simulink library "PC_Simulator_Lib"  (Simulink 8.2)
settings: Solver=ode45  StartTime=0.0  StopTime=10.0  RelTol=1e-3
values from neighbouring files (symbols this model uses):
  data = [r1 r2 r3 r4 L1 L2 L3 L4]    [strasse_Bedatung_HNI_ITI.m]
  distSameLane = 60    [InitialisationsEnv.m]
  eng_speed = [0 60 120 180 240 300 360 420 480 540 600 660 ... (101 elements, 1x101)]    [engine_table.mat]    (also in motor_parameter_calc.m = omega)
  Heading_init = 0    [Start.m]
  inertiaLateral = 25*(radiusWheel)^2    (= 4.129024)    [Start.m]
  laneWidth = 3.6    [InitialisationsEnv.m]    (also in strasse_Bedatung_HNI_ITI.m)
  omega_engine = [0.000000 150.000000 500.000000 1000.000000 1500.000000 2000.000000 2500.000000 3000.000000 3500.000000 4000.000000 4500.000000 5000.000000 5500.000000 6000.000000]    [friction_tables.m]
  omega_max = 6000    [engine_table.mat]    (also in motor_parameter_calc.m)
  omega_wheel = [0 20 40 60 80 100 122 143.7 164]    [friction_tables.m]
  para_Fellow_8_Points = ADAS.Fellow_8_Points    [ADAS_parameters.m]
  position_start_x = [x1 x2 x3 x4 x5 x6 x7]    [strasse_Bedatung_HNI_ITI.m]
  position_start_y = [y1 y2 y3 y4 y5 y6 y7]    [strasse_Bedatung_HNI_ITI.m]
  rad3rdLine = 57.2    [InitialisationsEnv.m]    (also in strasse_Bedatung_HNI_ITI.m)
  radiusWheel = 16*2.54/100    (= 0.4064)    [Start.m]
  s_values = [S1 S2 S3 S4 S5 S6 S7]    [strasse_Bedatung_HNI_ITI.m]
  segmentLimits = [segment1EndThirdLine                   segment2EndThirdLine                   segment3EndThirdLine                   segment4EndThirdLine                   segment5EndThirdLine                   segment6EndThirdLine                   segment7EndThirdLine                   segment8EndThirdLine                   ]    [InitialisationsEnv.m]    (also in strasse_Bedatung_HNI_ITI.m)
  setPosT = [-1.8 -5.4 -1.8 -5.4 -1.8 -5.4 -1.8 -5.4 -1.8 -5.4]    [InitialisationsEnv.m]
  torque = [297.089227105 300.997600937 304.800343044 308.497453426 312.088932082 315.574779014 318.95499422 322.229577701 325.398529457 328.461849487 331.419537793 334.271594373 ... (101 elements, 1x101)]    [engine_table.mat]    (also in motor_parameter_calc.m = g)
  Torque_lost = [0.000000 -8.777780 -15.000000 -26.800000 -29.600000 -32.700000 -35.900000 -39.300000 -42.800000 -46.500000 -50.300000 -54.300000 -58.500000 -62.800000 ]*0.6    [friction_tables.m]
  Torque_lost_wheel = [0.8 0.8 0.75 0.7 0.4 0.3 0.2 0.07 0.07]*0.2    [friction_tables.m]
  X_init = 0    [Start.m]
  Y_init = 1.8    [Start.m]
  Z_init = 0    [Start.m]
undefined symbols (not defined in the file or in its folder): Acc_Pedal, ADAS, Brake_Pedal, Joystick, Newton, Para, Raphson, Standard_Devices, Steering_Wheel_Angle, UDP_Protocol
libraries: simulink x43, rtwinlib x7, dspnetwork x2, simulink_extras x1, vrlib x1
(part 8 of 13)

== system PC_Simulator_Lib/Vehicle dynamics/velocity/to_tire ==
  angel_of_rotation_of_front_left_wheel : Inport
  angel_of_rotation_of_front_Right_wheel : Inport  Port=2
  velocity_at_wheels_in_X_mux(4) : Inport  Port=3
  velocity_at_wheels_in_Y_mux(4) : Inport  Port=4
  Demux : Demux
  Demux1 : Demux
  La{,1..7} (8 alike) : Product  RndMeth=Zero
  Mux1 : Mux
  Mux6 : Mux
  Sum1 : Sum  Inputs=+-
  Sum2 : Sum
  Sum3 : Sum  Inputs=+-
  Sum4 : Sum
  T1 : Trigonometry
  T2 : Trigonometry  Operator=cos
  T3 : Trigonometry  Operator=cos
  T4 : Trigonometry
  velocity_at_wheels_in_X_mux(4)final : Outport
  velocity_at_wheels_in_Y_mux(4)final : Outport  Port=2
  wires:
  velocity_at_wheels_in_X_mux(4)/1 -> Demux/1
  velocity_at_wheels_in_Y_mux(4)/1 -> Demux1/1
  Demux/3 -> Mux6/3
  Demux/4 -> Mux6/4
  Demux1/3 -> Mux1/3
  Demux1/4 -> Mux1/4
  Mux6/1 -> velocity_at_wheels_in_X_mux(4)final/1
  Mux1/1 -> velocity_at_wheels_in_Y_mux(4)final/1
  angel_of_rotation_of_front_left_wheel/1 -> T2/1, T4/1
  angel_of_rotation_of_front_Right_wheel/1 -> T3/1, T1/1
  Demux/1 -> La/1, La3/1, La4/1
  T2/1 -> La2/2, La/2
  La/1 -> Sum4/1
  Demux1/1 -> La2/1, La1/1
  T4/1 -> La3/2, La1/2
  La1/1 -> Sum4/2
  Sum4/1 -> Mux6/1
  La4/1 -> Sum2/1
  La7/1 -> Sum2/2
  Sum2/1 -> Mux6/2
  Demux1/2 -> La5/1, La7/1
  La2/1 -> Sum3/1
  La3/1 -> Sum3/2
  Sum3/1 -> Mux1/1
  La5/1 -> Sum1/1
  La6/1 -> Sum1/2
  Sum1/1 -> Mux1/2
  T3/1 -> La5/2, La4/2
  Demux/2 -> La6/1
  T1/1 -> La6/2, La7/2

== system PC_Simulator_Lib/Vehicle dynamics/velocity/velocity_at_Front_Left ==
  rate_of_change_Yaw_Angle : Inport
  longitudenal_velocity_Vx : Inport  Port=2
  Lateral_velocity_Vy : Inport  Port=3
  Divide : Product  Inputs=*/
  Length_CG_Front_Wheels : Constant  Value=Para.VD.Length_Front.v
  Product : Product  RndMeth=Zero
  Product1 : Product  RndMeth=Zero
  Rfl : Math  Operator=sqrt  SaturateOnIntegerOverflow=on
  Sum : Sum  Inputs=|++
  Sum1 : Sum  Inputs=|++
  Sum2 : Sum  Inputs=|++
  Sum3 : Sum  Inputs=|-+
  T1 : Trigonometry  Operator=cos
  T2 : Trigonometry
  ThetaFl : Trigonometry  Operator=atan
  Vfl/CG : Product  RndMeth=Zero
  Vfr/CGx : Product  RndMeth=Zero
  Vfr/CGy : Product  RndMeth=Zero
  Width_of_Car/2 : Constant  Value=Para.VD.Wheel_Base_Width.v/2
  pi : Constant  Value=pi
  velocity_at_Front_left_in_X : Outport
  velocity_at_Front_left_in_Y : Outport  Port=2
  wires:
  Lateral_velocity_Vy/1 -> Sum2/2
  Sum2/1 -> velocity_at_Front_left_in_Y/1
  longitudenal_velocity_Vx/1 -> Sum1/2
  Sum1/1 -> velocity_at_Front_left_in_X/1
  rate_of_change_Yaw_Angle/1 -> Vfl/CG/2
  Sum/1 -> Rfl/1
  Product/1 -> Sum/1
  Length_CG_Front_Wheels/1 -> Divide/1, Product/2, Product/1
  Width_of_Car/2/1 -> Divide/2, Product1/2, Product1/1
  Product1/1 -> Sum/2
  Rfl/1 -> Vfl/CG/1
  Divide/1 -> ThetaFl/1
  ThetaFl/1 -> Sum3/1
  Vfl/CG/1 -> Vfr/CGy/1, Vfr/CGx/1
  T2/1 -> Vfr/CGy/2
  T1/1 -> Vfr/CGx/2
  Sum3/1 -> T2/1, T1/1
  Vfr/CGx/1 -> Sum1/1
  Vfr/CGy/1 -> Sum2/1
  pi/1 -> Sum3/2

== system PC_Simulator_Lib/Vehicle dynamics/velocity/velocity_at_Front_Right ==
  rate_of_change_Yaw_Angle : Inport
  longitudenal_velocity_Vx : Inport  Port=2
  Lateral_velocity_Vy : Inport  Port=3
  Divide : Product  Inputs=*/
  Length_CG_Front_Wheels : Constant  Value=Para.VD.Length_Front.v
  Product : Product  RndMeth=Zero
  Product1 : Product  RndMeth=Zero
  Rfr : Math  Operator=sqrt  SaturateOnIntegerOverflow=on
  Sum : Sum  Inputs=|++
  Sum1 : Sum  Inputs=|++
  Sum2 : Sum  Inputs=|++
  ThetaFr : Trigonometry  Operator=atan
  ThetaFr1 : Trigonometry  Operator=cos
  ThetaFr2 : Trigonometry
  Vfr/CG : Product  RndMeth=Zero
  Vfr/CG1 : Product  RndMeth=Zero
  Vfr/CG2 : Product  RndMeth=Zero
  Width_of_Car/2 : Constant  Value=Para.VD.Wheel_Base_Width.v/2
  sign : Gain
  velocity_at_Front_Right_in_X : Outport
  velocity_at_Front_Right_in_Y : Outport  Port=2
  wires:
  Vfr/CG2/1 -> Sum2/1
  Vfr/CG1/1 -> Sum1/1
  sign/1 -> ThetaFr1/1, ThetaFr2/1
  ThetaFr1/1 -> Vfr/CG1/2
  ThetaFr2/1 -> Vfr/CG2/2
  Vfr/CG/1 -> Vfr/CG1/1, Vfr/CG2/1
  ThetaFr/1 -> sign/1
  Divide/1 -> ThetaFr/1
  Rfr/1 -> Vfr/CG/1
  Product1/1 -> Sum/2
  Width_of_Car/2/1 -> Product1/1, Product1/2, Divide/2
  Length_CG_Front_Wheels/1 -> Product/1, Product/2, Divide/1
  Product/1 -> Sum/1
  Sum/1 -> Rfr/1
  rate_of_change_Yaw_Angle/1 -> Vfr/CG/2
  Sum1/1 -> velocity_at_Front_Right_in_X/1
  longitudenal_velocity_Vx/1 -> Sum1/2
  Sum2/1 -> velocity_at_Front_Right_in_Y/1
  Lateral_velocity_Vy/1 -> Sum2/2

== system PC_Simulator_Lib/Vehicle dynamics/velocity/velocity_at_Rear_Left ==
  rate_of_change_Yaw_Angle : Inport
  longitudenal_velocity_Vx : Inport  Port=2
  Lateral_velocity_Vy : Inport  Port=3
  Divide : Product  Inputs=*/
  Divide1 : Product  Inputs=*/
  Length_CG_Rear_Wheels : Constant  Value=Para.VD.Length_Rear.v
  Product : Product  RndMeth=Zero
  Product1 : Product  RndMeth=Zero
  Rrl : Math  Operator=sqrt  SaturateOnIntegerOverflow=on
  Sum{,1..3} (4 alike) : Sum  Inputs=|++
  T1 : Trigonometry  Operator=cos
  T2 : Trigonometry
  Thetarl : Trigonometry  Operator=atan
  Vrl/CG : Product  RndMeth=Zero
  Vrl/CGx : Product  RndMeth=Zero
  Vrl/CGy : Product  RndMeth=Zero
  Width_of_Car/2 : Constant  Value=Para.VD.Wheel_Base_Width.v/2
  pi : Constant  Value=pi
  s : Trigonometry  Operator=atan
  velocity_at_Rear_left_in_X : Outport
  velocity_at_Rear_left_in_Y : Outport  Port=2
  slip_angel_at_Rear_left : Outport  Port=3
  wires:
  Vrl/CGy/1 -> Sum2/1
  Vrl/CGx/1 -> Sum1/1
  Sum3/1 -> T1/1, T2/1
  T1/1 -> Vrl/CGx/2
  T2/1 -> Vrl/CGy/2
  Vrl/CG/1 -> Vrl/CGx/1, Vrl/CGy/1
  Thetarl/1 -> Sum3/1
  Divide/1 -> Thetarl/1
  Rrl/1 -> Vrl/CG/1
  Product1/1 -> Sum/2
  Width_of_Car/2/1 -> Product1/1, Product1/2, Divide/2
  Length_CG_Rear_Wheels/1 -> Product/1, Product/2, Divide/1
  Product/1 -> Sum/1
  Sum/1 -> Rrl/1
  rate_of_change_Yaw_Angle/1 -> Vrl/CG/2
  Sum1/1 -> Divide1/2, velocity_at_Rear_left_in_X/1
  longitudenal_velocity_Vx/1 -> Sum1/2
  Sum2/1 -> Divide1/1, velocity_at_Rear_left_in_Y/1
  Lateral_velocity_Vy/1 -> Sum2/2
  pi/1 -> Sum3/2
  Divide1/1 -> s/1
  s/1 -> slip_angel_at_Rear_left/1

== system PC_Simulator_Lib/Vehicle dynamics/velocity/velocity_at_Rear_Right ==
  rate_of_change_Yaw_Angle : Inport
  longitudenal_velocity_Vx : Inport  Port=2
  Lateral_velocity_Vy : Inport  Port=3
  Divide : Product  Inputs=*/
  Length_CG_Rear_Wheels : Constant  Value=Para.VD.Length_Rear.v
  Product : Product  RndMeth=Zero
  Product1 : Product  RndMeth=Zero
  Rrr : Math  Operator=sqrt  SaturateOnIntegerOverflow=on
  Sum : Sum  Inputs=|++
  Sum1 : Sum  Inputs=|++
  Sum2 : Sum  Inputs=|++
  T1 : Trigonometry  Operator=cos
  T2 : Trigonometry
  Thetarr : Trigonometry  Operator=atan
  Vrr/CG : Product  RndMeth=Zero
  Vrr/CGx : Product  RndMeth=Zero
  Vrr/CGy : Product  RndMeth=Zero
  Width_of_Car/2 : Constant  Value=Para.VD.Wheel_Base_Width.v/2
  sign : Gain  Gain=-1
  velocity_at_Rear_Right_in_X : Outport
  velocity_at_Rear_Right_in_Y : Outport  Port=2
  wires:
  Lateral_velocity_Vy/1 -> Sum2/2
  Sum2/1 -> velocity_at_Rear_Right_in_Y/1
  longitudenal_velocity_Vx/1 -> Sum1/2
  Sum1/1 -> velocity_at_Rear_Right_in_X/1
  rate_of_change_Yaw_Angle/1 -> Vrr/CG/2
  Sum/1 -> Rrr/1
  Product/1 -> Sum/1
  Length_CG_Rear_Wheels/1 -> Divide/1, Product/2, Product/1
  Width_of_Car/2/1 -> Divide/2, Product1/2, Product1/1
  Product1/1 -> Sum/2
  Rrr/1 -> Vrr/CG/1
  Divide/1 -> Thetarr/1
  Thetarr/1 -> sign/1
  Vrr/CG/1 -> Vrr/CGy/1, Vrr/CGx/1
  T2/1 -> Vrr/CGy/2
  T1/1 -> Vrr/CGx/2
  sign/1 -> T2/1, T1/1
  Vrr/CGx/1 -> Sum1/1
  Vrr/CGy/1 -> Sum2/1

== system PC_Simulator_Lib/Vehicle dynamics/velocity/velocity_conditioning ==
  velocity_at_wheels_in_X_mux(4)in : Inport
  velocity_at_wheels_in_Y_mux(4)in : Inport  Port=2
  R_CGin : Inport  Port=3
  VxCG : Inport  Port=4
  VyCG : Inport  Port=5
  Constant1 : Constant  Value=eps
  Constant3 : Constant  Value=0
  Constant4 : Constant  Value=0
  Constant5 : Constant  Value=inf
  Demux : Demux
  Demux1 : Demux
  Logical Operator : Logic  Operator=NOT  AllPortsSameDT=off  OutDataTypeStr=boolean
  Logical Operator1 : Logic  Operator=OR  AllPortsSameDT=off  OutDataTypeStr=boolean
  Mux{1,4..6} (4 alike) : Mux
  Relational Operator1 : RelationalOperator  Operator===  OutDataTypeStr=boolean
  Relational Operator2 : RelationalOperator  Operator===  OutDataTypeStr=boolean
  Sum2 : Sum  Inputs=|++
  Switch1 : Switch
  Switch2 : Switch
  Switch3 : Switch
  Velocitytrim : Subsystem
  Velocitytrim1 : Subsystem
  Velocitytrim2 : Subsystem
  Velocitytrim3 : Subsystem
  Velocitytrim4 : Subsystem
  Velocitytrim5 : Subsystem
  Velocitytrim6 : Subsystem
  Velocitytrim7 : Subsystem
  velocity_at_wheels_in_X_mux(4)out : Outport
  velocity_at_wheels_in_Y_mux(4)out : Outport  Port=2
  R_CGout : Outport  Port=3
  wires:
  Constant3/1 -> Relational Operator1/2
  Constant4/1 -> Relational Operator2/2
  Relational Operator1/1 -> Logical Operator1/1
  Relational Operator2/1 -> Logical Operator1/2
  Mux5/1 -> Switch1/3
  Mux4/1 -> Switch2/3
  Constant5/1 -> Switch3/3
  Logical Operator/1 -> Switch1/2, Switch2/2, Switch3/2
  Logical Operator1/1 -> Logical Operator/1
  Switch3/1 -> Sum2/1
  Constant1/1 -> Sum2/2
  VxCG/1 -> Mux5/1, Mux5/2, Mux5/3, Mux5/4, Relational Operator1/1
  VyCG/1 -> Relational Operator2/1, Mux4/1, Mux4/2, Mux4/3, Mux4/4
  velocity_at_wheels_in_X_mux(4)in/1 -> Switch1/1
  velocity_at_wheels_in_Y_mux(4)in/1 -> Switch2/1
  R_CGin/1 -> Switch3/1
  Sum2/1 -> R_CGout/1
  Demux/1 -> Velocitytrim/1(vin)
  Demux/2 -> Velocitytrim1/1(vin)
  Demux/3 -> Velocitytrim2/1(vin)
  Demux/4 -> Velocitytrim3/1(vin)
  Velocitytrim/1(vout) -> Mux6/1
  Velocitytrim1/1(vout) -> Mux6/2
  Velocitytrim2/1(vout) -> Mux6/3
  Velocitytrim3/1(vout) -> Mux6/4
  Switch1/1 -> Demux/1
  Mux6/1 -> velocity_at_wheels_in_X_mux(4)out/1
  Demux1/1 -> Velocitytrim4/1(vin)
  Demux1/2 -> Velocitytrim5/1(vin)
  Demux1/3 -> Velocitytrim6/1(vin)
  Demux1/4 -> Velocitytrim7/1(vin)
  Velocitytrim4/1(vout) -> Mux1/1
  Velocitytrim5/1(vout) -> Mux1/2
  Velocitytrim6/1(vout) -> Mux1/3
  Velocitytrim7/1(vout) -> Mux1/4
  Mux1/1 -> velocity_at_wheels_in_Y_mux(4)out/1
  Switch2/1 -> Demux1/1

== system PC_Simulator_Lib/ADAS/Decision_Making_ADAS/Decision_Unit/critical_Braking_distance_determination ==
  v_relative_Sensor[m|s] : Inport
  1-D Lookup Table1 : Lookup_n-D  NumberOfTableDimensions=1  BreakpointsForDimension1=ADAS.EBA.Braking_Distance_LookUpTable.velocity  BeginIndexSearchUsingPreviousIndexResult=on  Table=ADAS.EBA.Braking_Distance_LookUpTable.Distance  InternalRulePriority=Speed  RndMeth=Simplest  InputSameDT=on
  Abs : Abs
  Divide : Product  Inputs=/**
  Gain : Gain  Gain=3.6
  Math Function : Math  Operator=square  SaturateOnIntegerOverflow=on
  Sign : Signum
  Unary Minus : UnaryMinus
  Braking_Distance[m] : Outport
  wires:
  v_relative_Sensor[m|s]/1 -> Abs/1, Sign/1, Math Function/1
  Math Function/1 -> Divide/2
  Divide/1 -> Braking_Distance[m]/1
  Gain/1 -> 1-D Lookup Table1/1
  1-D Lookup Table1/1 -> Divide/1
  Abs/1 -> Gain/1
  Sign/1 -> Unary Minus/1
  Unary Minus/1 -> Divide/3

== system PC_Simulator_Lib/ADAS/Decision_Making_ADAS/Maping_Input/signals_manipulation ==
  ACC_State : Inport
  Pilotiertes_Fahren_State : Inport  Port=2
  Emergency_Brkae_State : Inport  Port=3
  Emergency_Steering_State : Inport  Port=4
  Add : Sum  Inputs=++++
  Gain : Gain
  Gain1 : Gain  Gain=2
  Gain2 : Gain  Gain=3
  Gain3 : Gain  Gain=4
  Memory{1..4} (4 alike) : Memory
  Active_System : Outport
  wires:
  ACC_State/1 -> Memory1/1
  Pilotiertes_Fahren_State/1 -> Memory2/1
  Memory1/1 -> Gain/1
  Memory2/1 -> Gain1/1
  Add/1 -> Active_System/1
  Gain/1 -> Add/1
  Gain1/1 -> Add/2
  Emergency_Brkae_State/1 -> Memory3/1
  Memory3/1 -> Gain2/1
  Gain2/1 -> Add/3
  Gain3/1 -> Add/4
  Memory4/1 -> Gain3/1
  Emergency_Steering_State/1 -> Memory4/1

== system PC_Simulator_Lib/ADAS/Decision_Making_ADAS/Trajectory_calculatin_and_distance_control_and output_maping/Calculate_Desired_Trajectory ==
  Enable_Lateral_Controller : Inport
  T_Desired_initial[m] : Inport  Port=2
  Delta_T_Rate_limitl[m|s] : Inport  Port=3
  x[m] : Inport  Port=4
  y[m] : Inport  Port=5
  Yaw_Angle[rad] : Inport  Port=6
  Vx_CoG[m|s] : Inport  Port=7
  Velocity_Desired[m|s] : Inport  Port=8
  Bus Creator1 : BusCreator  Inputs=6
  Curvature_Calculation : Subsystem
  Gain{,1..5} (6 alike) : Gain
  Gain6 : Gain  Gain=pi/180
  Ground : Ground
  Road model ST_XY : Subsystem  Description=Simple road model to transform the (s,t) point of the local coordinate system to (x,y) point of the global coordinate system
  Scope1 : Scope
      settings: SaveName=ScopeData18
  Scope2 : Scope
  Scope3 : Scope  NumInputPorts=3
      settings: YMin=-5~-5~-5  YMax=5~5~5
  Strasse_xy : Subsystem
  Terminator : Terminator
  adding_Delta_s_and_road_restart : Subsystem
  applying_Desired_T_Gradually : Subsystem
  x_y_Virtual_Point_Calculation : Subsystem
  Desired_Track : Outport
  tag scope: T_VP=global
  wires:
  Bus Creator1/1 -> Desired_Track/1
  Gain3/1 -> Bus Creator1/4  "acceleration_Desired[m|s2]"
  Gain1/1 -> Bus Creator1/2  "y_Desired[m]"
  Gain4/1 -> Bus Creator1/5  "Heading_angle_Desired[rad]"
  Gain/1 -> Bus Creator1/1  "x_Desired[m]"
  Gain2/1 -> Bus Creator1/3  "Velocity_Desired[m|s]"
  Gain5/1 -> Bus Creator1/6  "Curvature_Desired_Track[1|m]"
  Gain6/1 -> Gain4/1
  Curvature_Calculation/1(Curvature_Given_Point[1|m]) -> Gain5/1
  x_y_Virtual_Point_Calculation/1(x_Virtual_Point[m]) -> Strasse_xy/1(x[m])
  x_y_Virtual_Point_Calculation/2(y_Virtual_Point[m]) -> Strasse_xy/2(y[m])
  Strasse_xy/1(s[m]) -> adding_Delta_s_and_road_restart/1(S_Virtual_Point_Actual[m])
  applying_Desired_T_Gradually/1(T_Desired_execute[m]) -> Scope1/1, Scope3/3, Road model ST_XY/2(t[m]), Curvature_Calculation/2(t_Value[m])
  adding_Delta_s_and_road_restart/1(S_Virtual_Point_Desired[m]) -> Road model ST_XY/1(s[m])
  Road model ST_XY/1(x[m]) -> Gain/1
  Road model ST_XY/2(y[m]) -> Gain1/1
  Road model ST_XY/3(headingAngle[deg]) -> Gain6/1
  Road model ST_XY/4(curvature[1/m]) -> Curvature_Calculation/1(Curvature_Road_Center[1|m])
  Strasse_xy/3(Heading_angle[rad]) -> Terminator/1
  Ground/1 -> Gain3/1
  Enable_Lateral_Controller/1 -> applying_Desired_T_Gradually/1(Enable_Lateral_Controller)
  T_Desired_initial[m]/1 -> applying_Desired_T_Gradually/3(T_Desired_initial[m]), Scope2/1, Scope3/2
  Delta_T_Rate_limitl[m|s]/1 -> applying_Desired_T_Gradually/4(Delta_T_Rate_limitl[m|s])
  Velocity_Desired[m|s]/1 -> Gain2/1
  Strasse_xy/2(t[m]) -> [T_VP], applying_Desired_T_Gradually/2(T_current[m]), Scope3/1
  Yaw_Angle[rad]/1 -> x_y_Virtual_Point_Calculation/3(Yaw_Angle[rad])
  x[m]/1 -> x_y_Virtual_Point_Calculation/1(x[m])
  y[m]/1 -> x_y_Virtual_Point_Calculation/2(y[m])
  Vx_CoG[m|s]/1 -> applying_Desired_T_Gradually/5(Vx_CoG[m|s]), adding_Delta_s_and_road_restart/2(Vx_CoG[m|s])

== system PC_Simulator_Lib/ADAS/Decision_Making_ADAS/Trajectory_calculatin_and_distance_control_and output_maping/Distance_Control ==
  Parameter_Bus : Inport
  Distance_2_Felow_Vehicle[m] : Inport  Port=2
  V_realtive[m|s] : Inport  Port=3
  V_Vehicle[m|s] : Inport  Port=4
  Time_Gap[s] : Inport  Port=5
  V_User_Set_Speed[m|s] : Inport  Port=6
  Enable : EnablePort
  Bus Selector : BusSelector  OutputSignals=acceleration_min[m|s2]
  Bus Selector1 : BusSelector  OutputSignals=V_Desired_max[m|s],V_Desired_min[m|s]
  Calculate_distances : Subsystem
  Distance controller : Subsystem
  V_Desired_Following[m|s] : Outport
  wires:
  V_Vehicle[m|s]/1 -> Distance controller/5(V_Vehicle[m|s]), Calculate_distances/3(V_Vehicle[m|s])
  Time_Gap[s]/1 -> Calculate_distances/4(Time_Gap_Desired[s])
  V_realtive[m|s]/1 -> Distance controller/4(V_realtive[m|s]), Calculate_distances/2(V_realtive[m|s])
  Distance controller/1(V_Desired_Following[m|s]) -> V_Desired_Following[m|s]/1
  Calculate_distances/1(S_Start_Braking[m]) -> Distance controller/2(S_Start_Braking[m])
  Distance_2_Felow_Vehicle[m]/1 -> Distance controller/1(Distance_2_Felow_Vehicle[m])
  Calculate_distances/2(Distance_Desired[m]) -> Distance controller/3(Distance_desired[m])
  Parameter_Bus/1 -> Bus Selector1/1, Bus Selector/1
  Bus Selector/1 -> Calculate_distances/1(acceleration_min[m|s2])  "<acceleration_min[m|s2]>"
  Bus Selector1/2 -> Distance controller/7(V_Desired_min[m|s])  "<V_Desired_min[m|s]>"
  Bus Selector1/1 -> Distance controller/6(V_Desired_max[m|s])  "<V_Desired_max[m|s]>"
  V_User_Set_Speed[m|s]/1 -> Distance controller/8(V_User_Set_Speed[m|s])

== system PC_Simulator_Lib/ADAS/Decision_Making_ADAS/Trajectory_calculatin_and_distance_control_and output_maping/Parameters ==
  Bus Creator : BusCreator
  Constant1 : Constant  Value=ADAS.Velocity_Control.a_min
  Constant2 : Constant  Value=200/3.6
  Constant3 : Constant  Value=0/3.6
  Constant4 : Constant  Value=ADAS.Velocity_Control.a_max
  Out1 : Outport
  wires:
  Bus Creator/1 -> Out1/1  "ADAS_Parameters"
  Constant4/1 -> Bus Creator/1  "acceleration_max[m|s2]"
  Constant1/1 -> Bus Creator/2  "acceleration_min[m|s2]"
  Constant2/1 -> Bus Creator/3  "V_Desired_max[m|s]"
  Constant3/1 -> Bus Creator/4  "V_Desired_min[m|s]"

== system PC_Simulator_Lib/ADAS/Execution_ADAS/Lateral_Controller_S_Function/Lateral_controller ==
  x_CoG_Global : Inport
  y_CoG_Global : Inport  Port=2
  v_CoG : Inport  Port=3
  Slip_Angle : Inport  Port=4
  Yaw_Angle : Inport  Port=5
  Yaw_Rate : Inport  Port=6
  x_Desire : Inport  Port=7
  y_Desired : Inport  Port=8
  Yaw_Desired : Inport  Port=9
  Yaw_Rate_Desired : Inport  Port=10
  v_Desired : Inport  Port=11
  a_Desired : Inport  Port=12
  Gain18 : Gain  Gain=-1
  Inverse_Steering_system : Subsystem
  control_law : Subsystem
  Steering_Wheel_Angle[norm] : Outport
  wires:
  Gain18/1 -> control_law/4(Slip_Angle)
  x_CoG_Global/1 -> control_law/1(x_CoG_Global)
  y_CoG_Global/1 -> control_law/2(y_CoG_Global)
  a_Desired/1 -> control_law/12(a_Desired)
  v_Desired/1 -> control_law/11(v_Desired)
  v_CoG/1 -> control_law/3(v_CoG)
  Yaw_Rate_Desired/1 -> control_law/10(Yaw_Rate_Desired)
  Slip_Angle/1 -> Gain18/1
  Yaw_Desired/1 -> control_law/9(Yaw_Desired)
  Yaw_Angle/1 -> control_law/5(Yaw_Angle)
  y_Desired/1 -> control_law/8(y_Desired)
  Yaw_Rate/1 -> control_law/6(Yaw_Rate)
  x_Desire/1 -> control_law/7(x_Desire)
  control_law/1(Inner_Wheel_Steeringangle[rad]) -> Inverse_Steering_system/1(Inner_Wheel_Steeringangle[rad])
  Inverse_Steering_system/1(Steering_Wheel_Angle[norm]) -> Steering_Wheel_Angle[norm]/1

== system PC_Simulator_Lib/ADAS/Execution_ADAS/Lateral_Controller_S_Function/calculate_slip_ange_and_absolute_velocity ==
  Vx_CoG[m|s] : Inport
  Vy_CoG[m|s] : Inport  Port=2
  Add : Sum
  Add1 : Sum
  Compare To Constant1 : simulink/Logic and Bit Operations/Compare To Constant  relop=>=  const=1  OutDataTypeStr=boolean
  Constant : Constant  Value=eps
  Data Type Conversion : DataTypeConversion
  Math Function : Math  Operator=square  SaturateOnIntegerOverflow=on
  Math Function1 : Math  Operator=square  SaturateOnIntegerOverflow=on
  Product1 : Product
  Sqrt : Sqrt  AlgorithmType=Newton-Raphson  SaturateOnIntegerOverflow=on
  Trigonometric Function : Trigonometry  Operator=atan2
  v_CoG[m|s] : Outport
  Slip_Angle[rad] : Outport  Port=2
  wires:
  Constant/1 -> Add1/2
  Sqrt/1 -> Compare To Constant1/1, Add1/1
  Add/1 -> Sqrt/1
  Math Function1/1 -> Add/2
  Math Function/1 -> Add/1
  Add1/1 -> v_CoG[m|s]/1
  Vx_CoG[m|s]/1 -> Trigonometric Function/2, Math Function/1
  Trigonometric Function/1 -> Product1/1
  Compare To Constant1/1 -> Data Type Conversion/1
  Data Type Conversion/1 -> Product1/2
  Product1/1 -> Slip_Angle[rad]/1
  Vy_CoG[m|s]/1 -> Trigonometric Function/1, Math Function1/1

== system PC_Simulator_Lib/ADAS/Execution_ADAS/Longitudinal_Controller/Acceleration_Control ==
  a_desired[m|s2] : Inport
  a_acctual[m|s2] : Inport  Port=2
  Vx_CoG[m|s] : Inport  Port=3
  omega_4_Wheels[rad|s] : Inport  Port=4
  Omega_Engine[rad|s] : Inport  Port=5
  Gearbox_Gear_Ratio : Inport  Port=6
  Differential_Gear_Ratio : Inport  Port=7
  Add : Sum
  Add1 : Sum  Inputs=-+
  Add2 : Sum
  Add3 : Sum  Inputs=-+
  Brake_Pedal_Calculation : Subsystem
  Divide : Product  Inputs=*//
  Ground : Ground
  PI_Controller_plus_antiwindup_For_Brake : Subsystem
  PI_Controller_plus_antiwindup_For_Trottel1 : Subsystem
  Saturation : Saturate  UpperLimit=1  LowerLimit=0
  Saturation1 : Saturate  UpperLimit=inf  LowerLimit=Para.DT.Fifth_Gear_reduction_Ratio.v
  Saturation2 : Saturate  UpperLimit=1  LowerLimit=0
  Throttel_angle_calculation : Subsystem
  Tractive_Force_Required_determination : Subsystem
  Wheel_Radius : Gain  Gain=radiusWheel
  Gas_Pedal[norm] : Outport
  Brake_Pedal[norm] : Outport  Port=2
  wires:
  a_desired[m|s2]/1 -> Tractive_Force_Required_determination/1(a_desired[m|s2]), PI_Controller_plus_antiwindup_For_Trottel1/1(a_desired[m|s2]), PI_Controller_plus_antiwindup_For_Brake/1(a_desired[m|s2])
  Ground/1 -> Tractive_Force_Required_determination/4(Road_inclination[rad])
  Vx_CoG[m|s]/1 -> Tractive_Force_Required_determination/2(Vx_CoG[m|s])
  omega_4_Wheels[rad|s]/1 -> Tractive_Force_Required_determination/3(omega_4_Wheels[rad|s])
  Tractive_Force_Required_determination/1(F_tire_required[N]) -> Wheel_Radius/1
  Wheel_Radius/1 -> Brake_Pedal_Calculation/1(Torque_Wheel_required[Nm]), Divide/1  "Torque_Wheel_required[Nm]"
  Gearbox_Gear_Ratio/1 -> Brake_Pedal_Calculation/3(Gearbox_Gear_Ratio), Saturation1/1
  Differential_Gear_Ratio/1 -> Brake_Pedal_Calculation/4(Differential_Gear_Ratio), Divide/3
  Divide/1 -> Throttel_angle_calculation/1(Torque_Engine_required[Nm])  "Torque_Engine_required[Nm]"
  Omega_Engine[rad|s]/1 -> Throttel_angle_calculation/2(Omega_Engine[rad|s]), Brake_Pedal_Calculation/2(Omega_Engine[rad|s])
  Saturation1/1 -> Divide/2
  Add/1 -> Saturation/1, Add1/1
  a_acctual[m|s2]/1 -> PI_Controller_plus_antiwindup_For_Trottel1/2(a_acctual[m|s2]), PI_Controller_plus_antiwindup_For_Brake/2(a_acctual[m|s2])
  PI_Controller_plus_antiwindup_For_Trottel1/1(Gas_Pedal_Zusatz[norm]) -> Add/2
  Saturation/1 -> Gas_Pedal[norm]/1, Add1/2
  Add1/1 -> PI_Controller_plus_antiwindup_For_Trottel1/3(Difference_on_sides_Saturation)
  Add2/1 -> Saturation2/1, Add3/1
  Saturation2/1 -> Brake_Pedal[norm]/1, Add3/2
  Add3/1 -> PI_Controller_plus_antiwindup_For_Brake/3(Difference_on_sides_Saturation)
  Brake_Pedal_Calculation/2(Brake_control_is_inactive[bool]) -> PI_Controller_plus_antiwindup_For_Trottel1/4(Brake_control_is_inactive[bool]), PI_Controller_plus_antiwindup_For_Brake/4(Brake_control_is_inactive[bool])
  PI_Controller_plus_antiwindup_For_Brake/1(Brake_Pedal_Zusatz[norm]) -> Add2/2
  Throttel_angle_calculation/1(throutle_angle[norm]) -> PI_Controller_plus_antiwindup_For_Trottel1/5(Gas_Pedal_Inverse_Motor[norm]), Add/1
  Brake_Pedal_Calculation/1(Brake_Pedal[norm]) -> Add2/1

== system PC_Simulator_Lib/ADAS/Execution_ADAS/Longitudinal_Controller/Velocity_Control ==
  Vx_desired[m|s] : Inport
  Vx_acctual[m|s] : Inport  Port=2
  acceleration_max[m|s2] : Inport  Port=3
  acceleration_min[m|s2] : Inport  Port=4
  Enable : EnablePort
  Add : Sum
  Add1 : Sum
  Integrator : Integrator
  Kb : Gain  Gain=ADAS.Velocity_Control.Kb
  Ki : Gain  Gain=ADAS.Velocity_Control.Ki
  Kp : Gain  Gain=ADAS.Velocity_Control.Kp
  Saturation Dynamic : simulink/Discontinuities/Saturation Dynamic  OutMin=[]  OutMax=[]  OutDataTypeStr=Inherit: Same as second input  OutDataType=fixdt(1, 16)  OutScaling=2^-10  DoSatur=off
  Subtract1 : Sum  Inputs=+-
  Subtract2 : Sum  Inputs=-+
  a_desired[m|s2] : Outport
  wires:
  Vx_desired[m|s]/1 -> Subtract1/1
  Vx_acctual[m|s]/1 -> Subtract1/2
  Subtract1/1 -> Kp/1, Ki/1
  Integrator/1 -> Add/2
  Kp/1 -> Add/1
  Add1/1 -> Integrator/1
  Ki/1 -> Add1/1
  Kb/1 -> Add1/2
  Subtract2/1 -> Kb/1
  Saturation Dynamic/1 -> a_desired[m|s2]/1, Subtract2/2
  Add/1 -> Saturation Dynamic/2, Subtract2/1
  acceleration_max[m|s2]/1 -> Saturation Dynamic/1
  acceleration_min[m|s2]/1 -> Saturation Dynamic/3

== system PC_Simulator_Lib/ADAS/Execution_ADAS/Output_Interface/Subsystem ==
  Acc_Pedal_ADAS[norm] : Inport
  Brake_Pedal__ADAS[norm] : Inport  Port=2
  Steering_Wheel_Angle_ADAS[norm] : Inport  Port=3
  Eanbel_Longitudidinal_Controller : Inport  Port=4
  Eanbel_Lateral_Controller : Inport  Port=5
  Acc_Pedal_user[norm] : Inport  Port=6
  Brake_Pedal_user[norm] : Inport  Port=7
  Steering_Wheel_Angle_User[norm] : Inport  Port=8
  Override_Longitudinal_Controller : Inport  Port=9
  Acc_Pedal_Decision_Unit_Override[norm] : Inport  Port=10
  Brake_Pedal_Decision_Unit_Override[norm] : Inport  Port=11
  Switch{,1..4} (5 alike) : Switch  Criteria=u2 > Threshold
  Acc_Pedal[norm] : Outport
  Brake_Pedal[norm] : Outport  Port=2
  Steering_Wheel_Angle[norm] : Outport  Port=3
  wires:
  Eanbel_Longitudidinal_Controller/1 -> Switch1/2, Switch/2
  Acc_Pedal_user[norm]/1 -> Switch/3
  Brake_Pedal_user[norm]/1 -> Switch1/3
  Steering_Wheel_Angle_User[norm]/1 -> Switch2/3
  Switch2/1 -> Steering_Wheel_Angle[norm]/1
  Eanbel_Lateral_Controller/1 -> Switch2/2
  Acc_Pedal_ADAS[norm]/1 -> Switch/1
  Steering_Wheel_Angle_ADAS[norm]/1 -> Switch2/1
  Brake_Pedal__ADAS[norm]/1 -> Switch1/1
  Switch/1 -> Acc_Pedal[norm]/1
  Switch3/1 -> ?
  Switch1/1 -> Brake_Pedal[norm]/1
  Switch4/1 -> ?
  Override_Longitudinal_Controller/1 -> Switch4/2, Switch3/2
  Acc_Pedal_Decision_Unit_Override[norm]/1 -> Switch3/1
  Brake_Pedal_Decision_Unit_Override[norm]/1 -> Switch4/1

== system PC_Simulator_Lib/ADAS/Sensors_ADAS/Front_Long_Range_Radar_Sensor/Coordinate_TRansformation_of_Fellows_Points_Plus_Calculation_Distances_And_Angles ==
  Objects_Dectected[bool] : Inport
  Apex_Pos_Global[m] : Inport  Port=2
  Oriantation_VUT_Vector[rad] : Inport  Port=3
  Position_Fellows[m] : Inport  Port=4
  Oriantation_Fellows[rad] : Inport  Port=5
  Demux : Demux  Outputs=3
  MATLAB Function : MATLAB Function  TreatAsAtomicUnit=on
  Terminator : Terminator
  Terminator1 : Terminator
  delta_s_Vector[m] : Outport
  Angle_Horizontal_Vector[rad] : Outport  Port=2
  Positon_of_detected_Points[m] : Outport  Port=3
  wires:
  Objects_Dectected[bool]/1 -> MATLAB Function/1(Objects_Dectected)
  Position_Fellows[m]/1 -> MATLAB Function/2(Position_Fellows)
  Oriantation_Fellows[rad]/1 -> MATLAB Function/3(Oriantation_Fellows)
  MATLAB Function/1(delta_s) -> delta_s_Vector[m]/1
  Apex_Pos_Global[m]/1 -> MATLAB Function/4(Apex_Pos_Global)
  MATLAB Function/2(Angle) -> Angle_Horizontal_Vector[rad]/1
  Oriantation_VUT_Vector[rad]/1 -> Demux/1
  Demux/3 -> MATLAB Function/5(yaw_VUT)
  Demux/1 -> Terminator/1
  Demux/2 -> Terminator1/1
  MATLAB Function/3(position) -> Positon_of_detected_Points[m]/1

== system PC_Simulator_Lib/ADAS/Sensors_ADAS/Front_Long_Range_Radar_Sensor/First_STage_Coordinate_Transformation ==
  Position_VUT_Vector[m] : Inport
  Oriantation_VUT_Vector[rad] : Inport  Port=2
  Position_Fellows[m] : Inport  Port=3
  Oriantation_Fellows[rad] : Inport  Port=4
  Bus to Vector : BusToVector
  Mux : Mux  Inputs=7
  Radar_Triangles_Transformation_From_Local2Global : Subsystem
  Triangles_2_Fellows_Coord_Transformation_Plus_Sphere_Filtering : Subsystem
  Upper_Triangles_Vector[m] : Outport
  Centeral_Triangles_Vector[m] : Outport  Port=2
  Lower_Triangles_Vector[m] : Outport  Port=3
  Inside_Sphere_Vector[bool] : Outport  Port=4
  Round_done[bool] : Outport  Port=5
  Apex_Position_Global[m] : Outport  Port=6
  wires:
  Radar_Triangles_Transformation_From_Local2Global/1(Apex_Position_Global_output[m]) -> Apex_Position_Global[m]/1
  Radar_Triangles_Transformation_From_Local2Global/9(Round_done[bool]) -> Round_done[bool]/1
  Oriantation_VUT_Vector[rad]/1 -> Radar_Triangles_Transformation_From_Local2Global/2(Oriantation_VUT_Vector[rad])
  Position_VUT_Vector[m]/1 -> Bus to Vector/1
  Radar_Triangles_Transformation_From_Local2Global/2(Apex_Position_Global[m]) -> Mux/1
  Radar_Triangles_Transformation_From_Local2Global/7(Lower_triangle_LeftPoint_Position_Global[m]) -> Mux/6
  Radar_Triangles_Transformation_From_Local2Global/8(Lower_triangle_RightPoint_Position_Global[m]) -> Mux/7
  Radar_Triangles_Transformation_From_Local2Global/6(Upper_triangle_RightPoint_Position_Global[m]) -> Mux/5
  Radar_Triangles_Transformation_From_Local2Global/4(Centeral_triangle_RightPoint_Position_Global[m]) -> Mux/3
  Radar_Triangles_Transformation_From_Local2Global/5(Upper_triangle_LeftPoint_Position_Global[m]) -> Mux/4
  Radar_Triangles_Transformation_From_Local2Global/3(Centeral_triangle_LeftPoint_Position_Global[m]) -> Mux/2
  Mux/1 -> Triangles_2_Fellows_Coord_Transformation_Plus_Sphere_Filtering/1(Triangels_Points_Glob[m])
  Bus to Vector/1 -> Radar_Triangles_Transformation_From_Local2Global/1(Position_VUT_Vector[m]), Triangles_2_Fellows_Coord_Transformation_Plus_Sphere_Filtering/2(Position_VUT_Vector[m])
  Triangles_2_Fellows_Coord_Transformation_Plus_Sphere_Filtering/1(Upper_Triangle_Vector[m]) -> Upper_Triangles_Vector[m]/1
  Triangles_2_Fellows_Coord_Transformation_Plus_Sphere_Filtering/2(Centeral_Triangle_Vector[m]) -> Centeral_Triangles_Vector[m]/1
  Triangles_2_Fellows_Coord_Transformation_Plus_Sphere_Filtering/4(Inside_Sphere_Vector[bool]) -> Inside_Sphere_Vector[bool]/1
  Triangles_2_Fellows_Coord_Transformation_Plus_Sphere_Filtering/3(Lower_Triangle_Vector[m]) -> Lower_Triangles_Vector[m]/1
  Position_Fellows[m]/1 -> Triangles_2_Fellows_Coord_Transformation_Plus_Sphere_Filtering/3(Position_Fellows[m])
  Oriantation_Fellows[rad]/1 -> Triangles_2_Fellows_Coord_Transformation_Plus_Sphere_Filtering/4(Oriantation_Fellows[rad])

== system PC_Simulator_Lib/ADAS/Sensors_ADAS/Front_Long_Range_Radar_Sensor/Intersection_Detection ==
  Cuboid_Dimentions_vector[m] : Inport
  Tiangle_upper_Points_Vetctor[m] : Inport  Port=2
  Tiangle_Center_Points_Vetctor[m] : Inport  Port=3
  Tiangle_Lower_Points_Vetctor[m] : Inport  Port=4
  Inside_Sphere_Vector[bool] : Inport  Port=5
  Round_done[bool] : Inport  Port=6
  S-Function : S-Function  FunctionName=IntersectionDetection  Parameters=para_num_fellow,para_filter_radius  EnableBusSupport=off
  Objects_Dectected[bool] : Outport
  wires:
  Round_done[bool]/1 -> S-Function/6
  S-Function/1 -> Objects_Dectected[bool]/1
  Tiangle_upper_Points_Vetctor[m]/1 -> S-Function/2
  Cuboid_Dimentions_vector[m]/1 -> S-Function/1
  Tiangle_Lower_Points_Vetctor[m]/1 -> S-Function/4
  Tiangle_Center_Points_Vetctor[m]/1 -> S-Function/3
  Inside_Sphere_Vector[bool]/1 -> S-Function/5

== system PC_Simulator_Lib/ADAS/Sensors_ADAS/Front_Mid_Range_Radar_Sensor/Coordinate_TRansformation_of_Fellows_Points_Plus_Calculation_Distances_And_Angles ==
  Objects_Dectected[bool] : Inport
  Apex_Pos_Global[m] : Inport  Port=2
  Oriantation_VUT_Vector[rad] : Inport  Port=3
  Position_Fellows[m] : Inport  Port=4
  Oriantation_Fellows[rad] : Inport  Port=5
  Demux : Demux  Outputs=3
  MATLAB Function : MATLAB Function  TreatAsAtomicUnit=on
  Terminator : Terminator
  Terminator1 : Terminator
  delta_s_Vector[m] : Outport
  Angle_Horizontal_Vector[rad] : Outport  Port=2
  Positon_of_detected_Points[m] : Outport  Port=3
  wires:
  Objects_Dectected[bool]/1 -> MATLAB Function/1(Objects_Dectected)
  Position_Fellows[m]/1 -> MATLAB Function/2(Position_Fellows)
  Oriantation_Fellows[rad]/1 -> MATLAB Function/3(Oriantation_Fellows)
  MATLAB Function/1(delta_s) -> delta_s_Vector[m]/1
  Apex_Pos_Global[m]/1 -> MATLAB Function/4(Apex_Pos_Global)
  MATLAB Function/2(Angle) -> Angle_Horizontal_Vector[rad]/1
  Oriantation_VUT_Vector[rad]/1 -> Demux/1
  Demux/3 -> MATLAB Function/5(yaw_VUT)
  Demux/1 -> Terminator/1
  Demux/2 -> Terminator1/1
  MATLAB Function/3(position) -> Positon_of_detected_Points[m]/1

== system PC_Simulator_Lib/ADAS/Sensors_ADAS/Front_Mid_Range_Radar_Sensor/First_STage_Coordinate_Transformation ==
  Position_VUT_Vector[m] : Inport
  Oriantation_VUT_Vector[rad] : Inport  Port=2
  Position_Fellows[m] : Inport  Port=3
  Oriantation_Fellows[rad] : Inport  Port=4
  Bus to Vector : BusToVector
  Mux : Mux  Inputs=7
  Radar_Triangles_Transformation_From_Local2Global : Subsystem
  Triangles_2_Fellows_Coord_Transformation_Plus_Sphere_Filtering : Subsystem
  Upper_Triangles_Vector[m] : Outport
  Centeral_Triangles_Vector[m] : Outport  Port=2
  Lower_Triangles_Vector[m] : Outport  Port=3
  Inside_Sphere_Vector[bool] : Outport  Port=4
  Round_simulation_time[ms] : Outport  Port=5
  Apex_Position_Global[m] : Outport  Port=6
  wires:
  Radar_Triangles_Transformation_From_Local2Global/1(Apex_Position_Global_output[m]) -> Apex_Position_Global[m]/1
  Radar_Triangles_Transformation_From_Local2Global/9(Round_simulation_time[ms]) -> Round_simulation_time[ms]/1
  Oriantation_VUT_Vector[rad]/1 -> Radar_Triangles_Transformation_From_Local2Global/2(Oriantation_VUT_Vector[rad])
  Position_VUT_Vector[m]/1 -> Bus to Vector/1
  Radar_Triangles_Transformation_From_Local2Global/2(Apex_Position_Global[m]) -> Mux/1
  Radar_Triangles_Transformation_From_Local2Global/7(Lower_triangle_LeftPoint_Position_Global[m]) -> Mux/6
  Radar_Triangles_Transformation_From_Local2Global/8(Lower_triangle_RightPoint_Position_Global[m]) -> Mux/7
  Radar_Triangles_Transformation_From_Local2Global/6(Upper_triangle_RightPoint_Position_Global[m]) -> Mux/5
  Radar_Triangles_Transformation_From_Local2Global/4(Centeral_triangle_RightPoint_Position_Global[m]) -> Mux/3
  Radar_Triangles_Transformation_From_Local2Global/5(Upper_triangle_LeftPoint_Position_Global[m]) -> Mux/4
  Radar_Triangles_Transformation_From_Local2Global/3(Centeral_triangle_LeftPoint_Position_Global[m]) -> Mux/2
  Mux/1 -> Triangles_2_Fellows_Coord_Transformation_Plus_Sphere_Filtering/1(Triangels_Points_Glob[m])
  Bus to Vector/1 -> Triangles_2_Fellows_Coord_Transformation_Plus_Sphere_Filtering/2(Position_VUT_Vector[m]), Radar_Triangles_Transformation_From_Local2Global/1(Position_VUT_Vector[m])
  Triangles_2_Fellows_Coord_Transformation_Plus_Sphere_Filtering/1(Upper_Triangle_Vector[m]) -> Upper_Triangles_Vector[m]/1
  Triangles_2_Fellows_Coord_Transformation_Plus_Sphere_Filtering/2(Centeral_Triangle_Vector[m]) -> Centeral_Triangles_Vector[m]/1
  Triangles_2_Fellows_Coord_Transformation_Plus_Sphere_Filtering/4(Inside_Sphere_Vector[bool]) -> Inside_Sphere_Vector[bool]/1
  Triangles_2_Fellows_Coord_Transformation_Plus_Sphere_Filtering/3(Lower_Triangle_Vector[m]) -> Lower_Triangles_Vector[m]/1
  Position_Fellows[m]/1 -> Triangles_2_Fellows_Coord_Transformation_Plus_Sphere_Filtering/3(Position_Fellows[m])
  Oriantation_Fellows[rad]/1 -> Triangles_2_Fellows_Coord_Transformation_Plus_Sphere_Filtering/4(Oriantation_Fellows[rad])

== system PC_Simulator_Lib/ADAS/Sensors_ADAS/Front_Mid_Range_Radar_Sensor/Intersection_Detection ==
  Cuboid_Dimentions_vector[m] : Inport
  Tiangle_upper_Points_Vetctor[m] : Inport  Port=2
  Tiangle_Center_Points_Vetctor[m] : Inport  Port=3
  Tiangle_Lower_Points_Vetctor[m] : Inport  Port=4
  Inside_Sphere_Vector[bool] : Inport  Port=5
  Round_simulation_time[ms] : Inport  Port=6
  S-Function : S-Function  FunctionName=IntersectionDetection  Parameters=para_num_fellow,para_filter_radius  EnableBusSupport=off
  Objects_Dectected[bool] : Outport
  wires:
  Round_simulation_time[ms]/1 -> S-Function/6
  S-Function/1 -> Objects_Dectected[bool]/1
  Tiangle_upper_Points_Vetctor[m]/1 -> S-Function/2
  Cuboid_Dimentions_vector[m]/1 -> S-Function/1
  Tiangle_Lower_Points_Vetctor[m]/1 -> S-Function/4
  Tiangle_Center_Points_Vetctor[m]/1 -> S-Function/3
  Inside_Sphere_Vector[bool]/1 -> S-Function/5

== system PC_Simulator_Lib/ADAS/Sensors_ADAS/Input_Maping/Fellows ==
  Feedback_Simulationsumgebung : Inport
  Bus Creator : BusCreator  Inputs=14
  Subsystem1 : Subsystem
  Subsystem2 : Subsystem
  Subsystem3 : Subsystem
  Subsystem4 : Subsystem
  Subsystem5 : Subsystem
  Position_Fellows[m] : Outport
  Oriantation_Fellows[rad] : Outport  Port=2
  wires:
  Subsystem2/10(Vehicle_10_Vector) -> Bus Creator/10
  Subsystem2/5(Vehicle_5_Vector) -> Bus Creator/5
  Subsystem2/7(Vehicle_7_Vector) -> Bus Creator/7
  Subsystem2/2(Vehicle_2_Vector) -> Bus Creator/2
  Subsystem2/8(Vehicle_8_Vector) -> Bus Creator/8
  Subsystem2/4(Vehicle_4_Vector3) -> Bus Creator/4
  Subsystem2/9(Vehicle_9_Vector) -> Bus Creator/9
  Subsystem2/3(Vehicle_3_Vector) -> Bus Creator/3
  Subsystem2/13(Vehicle_13_Vector) -> Bus Creator/13
  Subsystem2/14(Vehicle_14_Vector) -> Bus Creator/14
  Subsystem2/11(Vehicle_11_Vector) -> Bus Creator/11
  Subsystem2/1(Vehicle_1_Vector) -> Bus Creator/1
  Subsystem2/6(Vehicle_6_Vector) -> Bus Creator/6
  Subsystem2/12(Vehicle_12_Vector) -> Bus Creator/12
  Feedback_Simulationsumgebung/1 -> Subsystem2/1(FeedBack)
  Bus Creator/1 -> Subsystem4/1(Position_and_Oriantation_Fellows_Vector), Subsystem3/1(Position_and_Oriantation_Fellows_Vector), Subsystem5/1(Position_and_Oriantation_Fellows_Vector), Subsystem1/1(Position_and_Oriantation_Fellows_Vector)
  Subsystem5/1(Position_Fellows[m]) -> Position_Fellows[m]/1
  Subsystem1/1(Oriantation_Fellows[m]) -> Oriantation_Fellows[rad]/1

== system PC_Simulator_Lib/ADAS/Sensors_ADAS/Input_Maping/VUT ==
  Feedback_Simulationsumgebung : Inport
  Bus Creator1 : BusCreator  Inputs=3
  Bus Creator2 : BusCreator  Inputs=3
  Bus Selector : BusSelector  OutputSignals=Vehicle_Dynamics.position_CoG.x_CoG[m],Vehicle_Dynamics.position_CoG.y_CoG[m],Vehicle_Dynamics.position_CoG.z_CoG[m]
  Bus Selector1 : BusSelector  OutputSignals=Vehicle_Dynamics.Oriantation_CoG.Roll_Angle,Vehicle_Dynamics.Oriantation_CoG.Pitch_Angle,Vehicle_Dynamics.Oriantation_CoG.Yaw_Angle
  Gain{,1..5} (6 alike) : Gain
  Position_Global_VUT_Vector[m] : Outport
  Oriantation_VUT_Vector[rad] : Outport  Port=2
  wires:
  Bus Creator1/1 -> Position_Global_VUT_Vector[m]/1  "Position_Global_VUT_Vector[m]"
  Bus Creator2/1 -> Oriantation_VUT_Vector[rad]/1  "Oriantation_VUT_Vector[rad]"
  Feedback_Simulationsumgebung/1 -> Bus Selector1/1, Bus Selector/1
  Bus Selector/1 -> Gain/1  "<x_CoG[m]>"
  Bus Selector/2 -> Gain1/1  "<y_CoG[m]>"
  Bus Selector/3 -> Gain2/1  "<z_CoG[m]>"
  Gain/1 -> Bus Creator1/1  "x_CoG[m]"
  Gain1/1 -> Bus Creator1/2  "y_CoG[m"
  Gain2/1 -> Bus Creator1/3  "z_CoG[m"
  Bus Selector1/3 -> Gain5/1  "<Yaw_Angle>"
  Gain3/1 -> Bus Creator2/1  "Roll_VUT[rad]"
  Gain4/1 -> Bus Creator2/2  "Pitch_VUT[rad]"
  Gain5/1 -> Bus Creator2/3  "Yaw_VUT[rad]"
  Bus Selector1/1 -> Gain3/1  "<Roll_Angle>"
  Bus Selector1/2 -> Gain4/1  "<Pitch_Angle>"

== system PC_Simulator_Lib/Drive_Train/4_Wheels_drive_train_and_Brake/Brake/Subsystem ==
  Torque_Brake_Nm : Inport
  Omega_rad/s : Inport  Port=2
  Compare To Constant : simulink/Logic and Bit Operations/Compare To Constant  relop=>=  const=0.1  OutDataTypeStr=uint8
  Compare To Constant1 : simulink/Logic and Bit Operations/Compare To Constant  relop=<=  const=-0.1  OutDataTypeStr=uint8
  Data Type Conversion : DataTypeConversion
  Logical Operator : Logic  Operator=OR  AllPortsSameDT=off  OutDataTypeStr=boolean
  Product : Product  Inputs=3  RndMeth=Zero
  Rate Limiter1 : RateLimiter  SampleTimeMode=inherited
  Sign : Signum
  Torque_Brake_act_Nm : Outport
  wires:
  Rate Limiter1/1 -> Product/3
  Compare To Constant1/1 -> Logical Operator/2
  Logical Operator/1 -> Data Type Conversion/1
  Data Type Conversion/1 -> Rate Limiter1/1
  Compare To Constant/1 -> Logical Operator/1
  Sign/1 -> Product/2
  Product/1 -> Torque_Brake_act_Nm/1
  Omega_rad/s/1 -> Sign/1, Compare To Constant/1, Compare To Constant1/1
  Torque_Brake_Nm/1 -> Product/1

== system PC_Simulator_Lib/Drive_Train/4_Wheels_drive_train_and_Brake/Brake/Subsystem1 ==
  v_X_CoG[m|s] : Inport
  Brake_Pedal[norm] : Inport  Port=2
  Compare To Constant : simulink/Logic and Bit Operations/Compare To Constant  relop=<  const=0.7  OutDataTypeStr=uint8
  Compare To Constant1 : simulink/Logic and Bit Operations/Compare To Constant  relop=>  const=-1  OutDataTypeStr=uint8
  Compare To Constant2 : simulink/Logic and Bit Operations/Compare To Constant  relop=>=  const=0.01  OutDataTypeStr=uint8
  Compare To Constant3 : simulink/Logic and Bit Operations/Compare To Constant  relop=<  const=-0.1  OutDataTypeStr=uint8
  Constant : Constant  Value=0
  Constant1 : Constant  Value=3.5
  Constant2 : Constant
  Data Type Conversion : DataTypeConversion
  Gain1 : Gain  Gain=-100
  Logical Operator : Logic  Inputs=3  AllPortsSameDT=off  OutDataTypeStr=boolean
  Logical Operator1 : Logic  AllPortsSameDT=off  OutDataTypeStr=boolean
  Product : Product  Inputs=3
  Subtract : Sum  Inputs=+-
  Switch : Switch  Criteria=u2 > Threshold
  Out1 : Outport
  wires:
  v_X_CoG[m|s]/1 -> Compare To Constant3/1, Compare To Constant1/1, Compare To Constant/1, Subtract/2
  Constant/1 -> Subtract/1
  Subtract/1 -> Gain1/1
  Gain1/1 -> Product/1
  Product/1 -> Out1/1
  Compare To Constant/1 -> Logical Operator/1
  Compare To Constant1/1 -> Logical Operator1/1, Logical Operator/2
  Logical Operator/1 -> Data Type Conversion/1
  Data Type Conversion/1 -> Product/2
  Compare To Constant2/1 -> Logical Operator/3
  Brake_Pedal[norm]/1 -> Compare To Constant2/1
  Compare To Constant3/1 -> Logical Operator1/2
  Logical Operator1/1 -> Switch/2
  Constant1/1 -> Switch/1
  Switch/1 -> Product/3
  Constant2/1 -> Switch/3

== system PC_Simulator_Lib/Drive_Train/4_Wheels_drive_train_and_Brake/FL/Alpha_Kappa_Selector2 ==
  Vx : Inport
  Vy : Inport  Port=2
  omega : Inport  Port=3
  Rdyn : Inport  Port=4
  Fx : Inport  Port=5
  Dynamik Anteil2 : Subsystem
  Saturation : Saturate  UpperLimit=1  LowerLimit=-1
  alpha_calc : Subsystem
  kappa : Outport
  alpha : Outport  Port=2
  wires:
  Fx/1 -> Dynamik Anteil2/1(Fx)
  Dynamik Anteil2/1(k) -> Saturation/1
  Saturation/1 -> kappa/1
  Rdyn/1 -> Dynamik Anteil2/4(R)
  omega/1 -> Dynamik Anteil2/3(omega)
  alpha_calc/1(alpha) -> alpha/1
  Vx/1 -> alpha_calc/2(Vx), Dynamik Anteil2/2(Vx)
  Vy/1 -> alpha_calc/1(Vy)

== system PC_Simulator_Lib/Drive_Train/4_Wheels_drive_train_and_Brake/FL/Wheel dynamics ==
  F_x : Inport
  Torque_Drive_Nm : Inport  Port=2
  Torque_Brake_Nm : Inport  Port=3
  Add : Sum  Inputs=++--
  Friction : Subsystem
  Gain : Gain  Gain=radiusWheel
  Gain1 : Gain  Gain=-1
  Gain2 : Gain  Gain=1/(inertiaLateral/2)
  Integrator : Integrator
  Subsystem : Subsystem
  Terminator : Terminator
  omega_radPs : Outport
  omegaDot_radPs2 : Outport  Port=2
  wires:
  Gain/1 -> Gain1/1
  F_x/1 -> Gain/1
  Gain1/1 -> Add/1
  Torque_Drive_Nm/1 -> Add/2
  Add/1 -> Gain2/1
  Gain2/1 -> Integrator/1, omegaDot_radPs2/1
  Integrator/1 -> omega_radPs/1, Friction/1(omega_radPs), Subsystem/2(Omega_rad/s)
  Friction/1(Torque_friction) -> Add/3
  Torque_Brake_Nm/1 -> Subsystem/1(Torque_Brake_Nm), Add/4
  Subsystem/1(Torque_Brake_act_Nm) -> Terminator/1

== system PC_Simulator_Lib/Drive_Train/4_Wheels_drive_train_and_Brake/FR/Alpha_Kappa_Selector2 ==
  Vx : Inport
  Vy : Inport  Port=2
  omega : Inport  Port=3
  Rdyn : Inport  Port=4
  Fx : Inport  Port=5
  Dynamik Anteil2 : Subsystem
  Saturation : Saturate  UpperLimit=1  LowerLimit=-1
  alpha_calc : Subsystem
  kappa : Outport
  alpha : Outport  Port=2
  wires:
  Fx/1 -> Dynamik Anteil2/1(Fx)
  Dynamik Anteil2/1(k) -> Saturation/1
  Saturation/1 -> kappa/1
  Rdyn/1 -> Dynamik Anteil2/4(R)
  omega/1 -> Dynamik Anteil2/3(omega)
  alpha_calc/1(alpha) -> alpha/1
  Vx/1 -> alpha_calc/2(Vx), Dynamik Anteil2/2(Vx)
  Vy/1 -> alpha_calc/1(Vy)

== system PC_Simulator_Lib/Drive_Train/4_Wheels_drive_train_and_Brake/FR/Wheel dynamics ==
  F_x : Inport
  Torque_Drive_Nm : Inport  Port=2
  Torque_Brake_Nm : Inport  Port=3
  Add : Sum  Inputs=++--
  Friction : Subsystem
  Gain : Gain  Gain=radiusWheel
  Gain1 : Gain  Gain=-1
  Gain2 : Gain  Gain=1/(inertiaLateral/2)
  Integrator : Integrator
  Subsystem : Subsystem
  Terminator : Terminator
  omega_radPs : Outport
  omegaDot_radPs2 : Outport  Port=2
  wires:
  Gain/1 -> Gain1/1
  F_x/1 -> Gain/1
  Gain1/1 -> Add/1
  Torque_Drive_Nm/1 -> Add/2
  Add/1 -> Gain2/1
  Gain2/1 -> Integrator/1, omegaDot_radPs2/1
  Integrator/1 -> omega_radPs/1, Friction/1(omega_radPs), Subsystem/2(Omega_rad/s)
  Friction/1(Torque_friction) -> Add/3
  Torque_Brake_Nm/1 -> Subsystem/1(Torque_Brake_Nm), Add/4
  Subsystem/1(Torque_Brake_act_Nm) -> Terminator/1

== system PC_Simulator_Lib/Drive_Train/4_Wheels_drive_train_and_Brake/RL/Alpha_Kappa_Selector2 ==
  Vx : Inport
  Vy : Inport  Port=2
  omega : Inport  Port=3
  Rdyn : Inport  Port=4
  Fx : Inport  Port=5
  Dynamik Anteil2 : Subsystem
  Saturation : Saturate  UpperLimit=1  LowerLimit=-1
  alpha_calc : Subsystem
  kappa : Outport
  alpha : Outport  Port=2
  wires:
  Fx/1 -> Dynamik Anteil2/1(Fx)
  Dynamik Anteil2/1(k) -> Saturation/1
  Saturation/1 -> kappa/1
  Rdyn/1 -> Dynamik Anteil2/4(R)
  omega/1 -> Dynamik Anteil2/3(omega)
  alpha_calc/1(alpha) -> alpha/1
  Vx/1 -> alpha_calc/2(Vx), Dynamik Anteil2/2(Vx)
  Vy/1 -> alpha_calc/1(Vy)

== system PC_Simulator_Lib/Drive_Train/4_Wheels_drive_train_and_Brake/RL/Wheel dynamics ==
  F_x : Inport
  Torque_Drive_Nm : Inport  Port=2
  Torque_Brake_Nm : Inport  Port=3
  Add : Sum  Inputs=++--
  Friction : Subsystem
  Gain : Gain  Gain=radiusWheel
  Gain1 : Gain  Gain=-1
  Gain2 : Gain  Gain=1/(inertiaLateral/2)
  Integrator : Integrator
  Subsystem : Subsystem
  Terminator : Terminator
  omega_radPs : Outport
  omegaDot_radPs2 : Outport  Port=2
  wires:
  Gain/1 -> Gain1/1
  F_x/1 -> Gain/1
  Gain1/1 -> Add/1
  Torque_Drive_Nm/1 -> Add/2
  Add/1 -> Gain2/1
  Gain2/1 -> Integrator/1, omegaDot_radPs2/1
  Integrator/1 -> omega_radPs/1, Friction/1(omega_radPs), Subsystem/2(Omega_rad/s)
  Friction/1(Torque_friction) -> Add/3
  Torque_Brake_Nm/1 -> Subsystem/1(Torque_Brake_Nm), Add/4
  Subsystem/1(Torque_Brake_act_Nm) -> Terminator/1

== system PC_Simulator_Lib/Drive_Train/4_Wheels_drive_train_and_Brake/RR/Alpha_Kappa_Selector2 ==
  Vx : Inport
  Vy : Inport  Port=2
  omega : Inport  Port=3
  Rdyn : Inport  Port=4
  Fx : Inport  Port=5
  Dynamik Anteil2 : Subsystem
  Saturation : Saturate  UpperLimit=1  LowerLimit=-1
  alpha_calc : Subsystem
  kappa : Outport
  alpha : Outport  Port=2
  wires:
  Fx/1 -> Dynamik Anteil2/1(Fx)
  Dynamik Anteil2/1(k) -> Saturation/1
  Saturation/1 -> kappa/1
  Rdyn/1 -> Dynamik Anteil2/4(R)
  omega/1 -> Dynamik Anteil2/3(omega)
  alpha_calc/1(alpha) -> alpha/1
  Vx/1 -> alpha_calc/2(Vx), Dynamik Anteil2/2(Vx)
  Vy/1 -> alpha_calc/1(Vy)

== system PC_Simulator_Lib/Drive_Train/4_Wheels_drive_train_and_Brake/RR/Wheel dynamics ==
  F_x : Inport
  Torque_Drive_Nm : Inport  Port=2
  Torque_Brake_Nm : Inport  Port=3
  Add : Sum  Inputs=++--
  Friction : Subsystem
  Gain : Gain  Gain=radiusWheel
  Gain1 : Gain  Gain=-1
  Gain2 : Gain  Gain=1/(inertiaLateral/2)
  Integrator : Integrator
  Subsystem : Subsystem
  Terminator : Terminator
  omega_radPs : Outport
  omegaDot_radPs2 : Outport  Port=2
  wires:
  Gain/1 -> Gain1/1
  F_x/1 -> Gain/1
  Gain1/1 -> Add/1
  Torque_Drive_Nm/1 -> Add/2
  Add/1 -> Gain2/1
  Gain2/1 -> Integrator/1, omegaDot_radPs2/1
  Integrator/1 -> omega_radPs/1, Friction/1(omega_radPs), Subsystem/2(Omega_rad/s)
  Friction/1(Torque_friction) -> Add/3
  Torque_Brake_Nm/1 -> Subsystem/1(Torque_Brake_Nm), Add/4
  Subsystem/1(Torque_Brake_act_Nm) -> Terminator/1
